simulink model "mask"  (R2014a)
settings: Solver=ode45  StartTime=0.0  StopTime=10.0  RelTol=1e-3
settings Model: Creator=pmi1kor  LastModifiedBy=ladmin
settings DebuggingCC: MergeDetectMultiDrivingBlocksExec=error

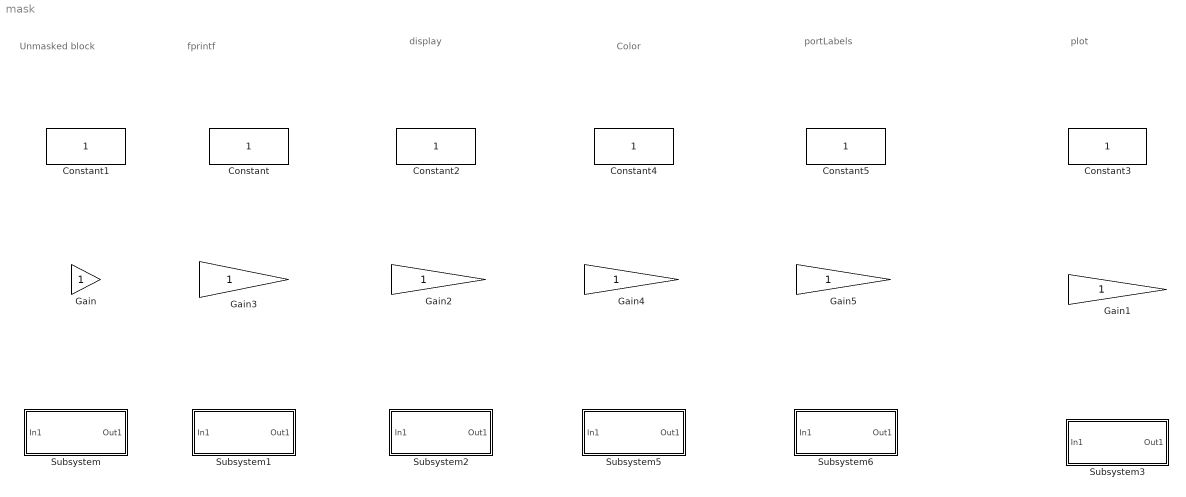
== system mask ==
  note: Unmasked block
  note: fprintf
  note: display
  note: plot
  note: Color
  note: portLabels
  Constant{,1..5} (6 alike) : Constant
      Constant mask Display: fprintf('fprintf label');
      Constant2 mask Display: disp('display label');
      Constant3 mask Display: plot(sin(0:3.14))
      Constant4 mask Display:
      | color('red')
      | disp('display label');
      Constant5 mask Display: port_label('output',1,'ehb port')
  Gain{,1..5} (6 alike) : Gain
      Gain1 mask Display: plot(sin(0:3.14))
      Gain2 mask Display: disp('display label')
      Gain3 mask Display: fprintf('fprintf label')
      Gain4 mask Display:
      | color('red')
      | disp('display label')
      Gain5 mask Display:
      | port_label('input',1,'ehb_in')
      | port_label('output',1,'ehb_out')
  Subsystem : Subsystem
  Subsystem1 : Subsystem
      mask Display: fprintf('fprintf label');
  Subsystem2 : Subsystem
      mask Display: disp('display label')
  Subsystem3 : Subsystem
      mask Display: plot(sin(0:3.14))
  Subsystem5 : Subsystem
      mask Display:
      | color('red')
      | disp('display label')
  Subsystem6 : Subsystem
      mask Display:
      | port_label('input',1,'ehb_in')
      | port_label('output',1,'ehb_out')

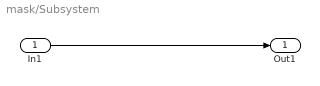
== system mask/Subsystem ==
  In1 : Inport
  Out1 : Outport
  wires:
  In1/1 -> Out1/1

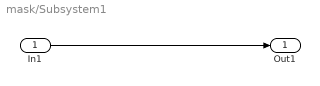
== system mask/Subsystem1 ==
  In1 : Inport
  Out1 : Outport
  wires:
  In1/1 -> Out1/1

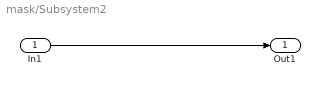
== system mask/Subsystem2 ==
  In1 : Inport
  Out1 : Outport
  wires:
  In1/1 -> Out1/1

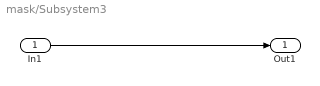
== system mask/Subsystem3 ==
  In1 : Inport
  Out1 : Outport
  wires:
  In1/1 -> Out1/1

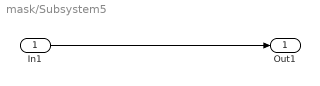
== system mask/Subsystem5 ==
  In1 : Inport
  Out1 : Outport
  wires:
  In1/1 -> Out1/1

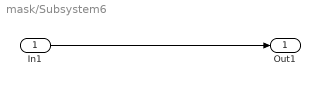
== system mask/Subsystem6 ==
  In1 : Inport
  Out1 : Outport
  wires:
  In1/1 -> Out1/1
